simulink model "nomonly"  (R2016b)
settings: Solver=VariableStepAuto  StartTime=0.0  StopTime=10.0  RelTol=1e-3
settings Model: Creator=root  LastModifiedBy=root

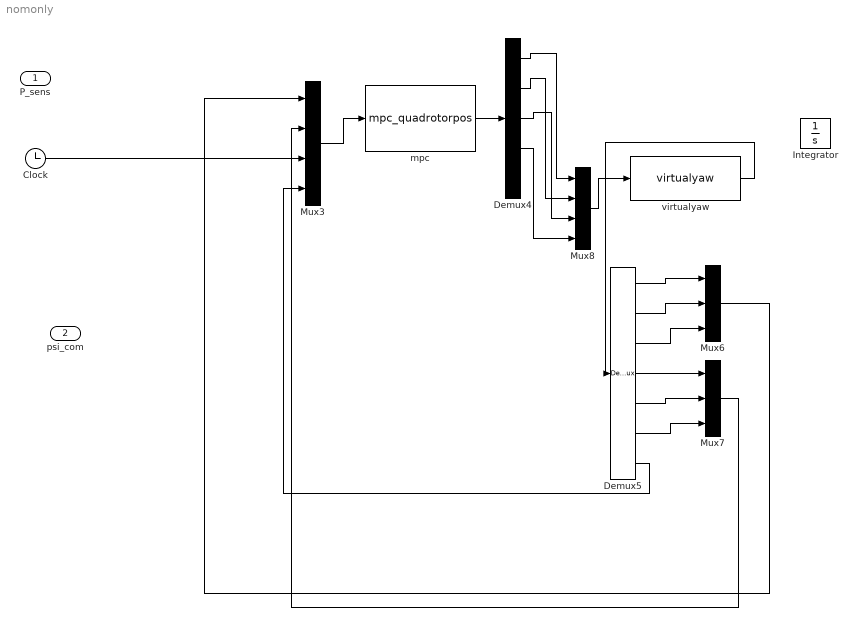
== system nomonly ==
  P_sens : Inport
  psi_com : Inport  Port=2
  Clock : Clock
  Demux4 : Demux  Outputs=5
  Demux5 : Demux  Outputs=7
  Integrator : Integrator
  Mux3 : Mux
  Mux6 : Mux  Inputs=3
  Mux7 : Mux  Inputs=3
  Mux8 : Mux
  mpc : MATLABFcn  MATLABFcn=mpc_quadrotorpos  OutputDimensions=5
  virtualyaw : S-Function  FunctionName=virtualyaw  SFunctionDeploymentMode=off  EnableBusSupport=off
  wires:
  Mux3/1 -> mpc/1
  Clock/1 -> Mux3/3
  mpc/1 -> Demux4/1
  Demux4/2 -> Mux8/2
  Demux4/1 -> Mux8/1
  Demux4/3 -> Mux8/3
  Demux5/1 -> Mux6/1
  Demux5/2 -> Mux6/2
  Demux5/3 -> Mux6/3
  Demux5/4 -> Mux7/1
  Demux5/5 -> Mux7/2
  Demux5/6 -> Mux7/3
  virtualyaw/1 -> Demux5/1
  Mux6/1 -> Mux3/1
  Mux7/1 -> Mux3/2
  Demux5/7 -> Mux3/4
  Demux4/4 -> Mux8/4
  Mux8/1 -> virtualyaw/1
